simulink subsystem "Vehicle_Navigation"  (R2020b)
settings: Solver=VariableStepAuto  StartTime=0.0  StopTime=10.0  RelTol=1e-3
libraries: simulink_extras x1
settings Model: Creator=rthom  LastModifiedBy=david

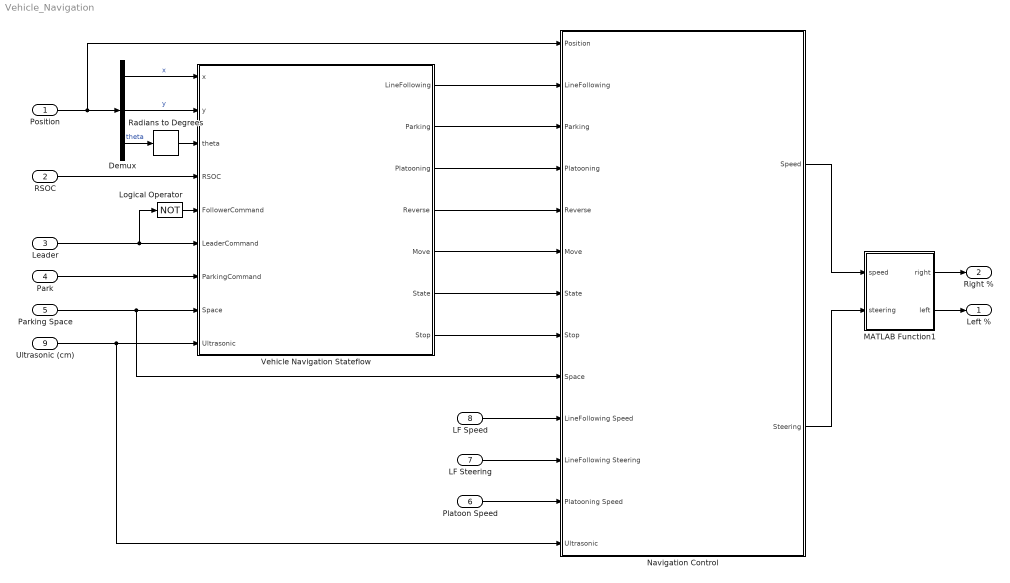
== system Vehicle_Navigation ==
  Position : Inport
  RSOC : Inport  Port=2
  Leader : Inport  Port=3
  Park : Inport  Port=4
  Parking Space : Inport  Port=5
  Platoon Speed : Inport  Port=6
  LF Steering : Inport  Port=7
  LF Speed : Inport  Port=8
  Ultrasonic (cm) : Inport  Port=9
  Demux : Demux  Outputs=3
  Logical Operator : Logic  Operator=NOT  AllPortsSameDT=off  OutDataTypeStr=boolean
  MATLAB Function1 : MATLAB Function  TreatAsAtomicUnit=on
  Navigation Control : Subsystem
  Radians to Degrees : simulink_extras/Transformations/Radians to Degrees
  Vehicle Navigation Stateflow : Stateflow chart  TreatAsAtomicUnit=on
  Left % : Outport
  Right % : Outport  Port=2
  wires:
  MATLAB Function1/1(right) -> Right %/1
  MATLAB Function1/2(left) -> Left %/1
  RSOC/1 -> Vehicle Navigation Stateflow/4(RSOC)
  Position/1 -> Demux/1, Navigation Control/1(Position)
  LF Speed/1 -> Navigation Control/10(LineFollowing Speed)
  Vehicle Navigation Stateflow/3(Platooning) -> Navigation Control/4(Platooning)
  Navigation Control/2(Steering) -> MATLAB Function1/2(steering)
  LF Steering/1 -> Navigation Control/11(LineFollowing Steering)
  Vehicle Navigation Stateflow/6(State) -> Navigation Control/7(State)
  Vehicle Navigation Stateflow/7(Stop) -> Navigation Control/8(Stop)
  Vehicle Navigation Stateflow/4(Reverse) -> Navigation Control/5(Reverse)
  Leader/1 -> Vehicle Navigation Stateflow/6(LeaderCommand), Logical Operator/1
  Vehicle Navigation Stateflow/1(LineFollowing) -> Navigation Control/2(LineFollowing)
  Vehicle Navigation Stateflow/2(Parking) -> Navigation Control/3(Parking)
  Demux/3 -> Radians to Degrees/1  "theta"
  Ultrasonic (cm)/1 -> Navigation Control/13(Ultrasonic), Vehicle Navigation Stateflow/9(Ultrasonic)
  Parking Space/1 -> Navigation Control/9(Space), Vehicle Navigation Stateflow/8(Space)
  Park/1 -> Vehicle Navigation Stateflow/7(ParkingCommand)
  Demux/2 -> Vehicle Navigation Stateflow/2(y)  "y"
  Platoon Speed/1 -> Navigation Control/12(Platooning Speed)
  Demux/1 -> Vehicle Navigation Stateflow/1(x)  "x"
  Vehicle Navigation Stateflow/5(Move) -> Navigation Control/6(Move)
  Navigation Control/1(Speed) -> MATLAB Function1/1(speed)
  Radians to Degrees/1 -> Vehicle Navigation Stateflow/3(theta)
  Logical Operator/1 -> Vehicle Navigation Stateflow/5(FollowerCommand)

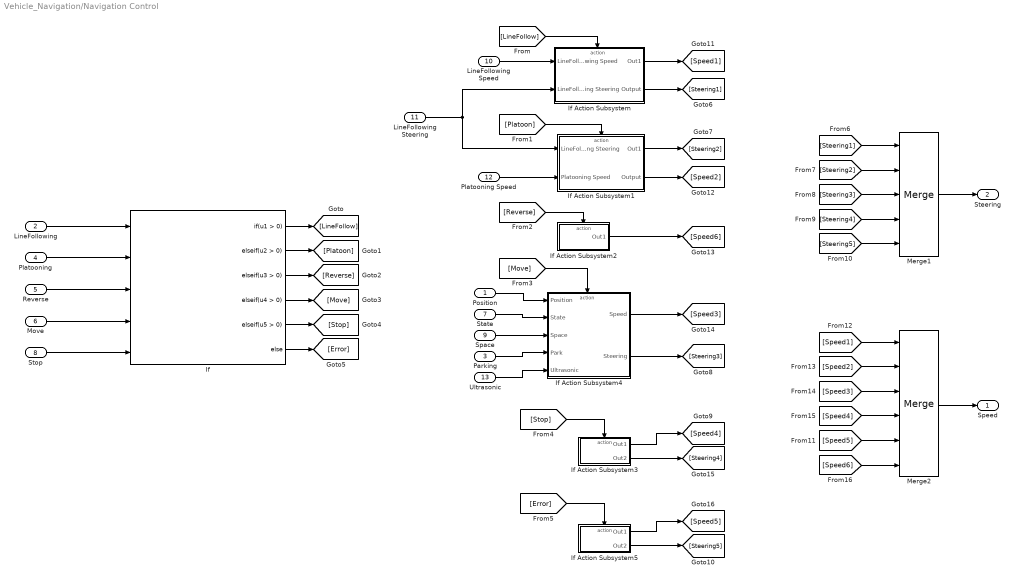
== system Vehicle_Navigation/Navigation Control ==
  Position : Inport
  LineFollowing : Inport  Port=2
  Parking : Inport  Port=3
  Platooning : Inport  Port=4
  Reverse : Inport  Port=5
  Move : Inport  Port=6
  State : Inport  Port=7
  Stop : Inport  Port=8
  Space : Inport  Port=9
  LineFollowing Speed : Inport  Port=10
  LineFollowing Steering : Inport  Port=11
  Platooning Speed : Inport  Port=12
  Ultrasonic : Inport  Port=13
  If : If  NumInputs=5  ElseIfExpressions=u2 > 0,u3 > 0,u4 > 0,u5 > 0
  If Action Subsystem : Subsystem  TreatAsAtomicUnit=on
  If Action Subsystem1 : Subsystem  TreatAsAtomicUnit=on
  If Action Subsystem2 : Subsystem  TreatAsAtomicUnit=on
  If Action Subsystem3 : Subsystem  TreatAsAtomicUnit=on
  If Action Subsystem4 : Subsystem  TreatAsAtomicUnit=on
  If Action Subsystem5 : Subsystem  TreatAsAtomicUnit=on
  Merge1 : Merge  Inputs=5
  Merge2 : Merge  Inputs=6
  Speed : Outport
  Steering : Outport  Port=2
  wires:
  Ultrasonic/1 -> If Action Subsystem4/5(Ultrasonic)
  Parking/1 -> If Action Subsystem4/4(Park)
  [Speed6] -> Merge2/6
  Merge2/1 -> Speed/1
  [Speed3] -> Merge2/3
  [Speed5] -> Merge2/5
  [Speed1] -> Merge2/1
  [Speed2] -> Merge2/2
  [Speed4] -> Merge2/4
  If Action Subsystem5/2(Out2) -> [Steering5]
  If Action Subsystem5/1(Out1) -> [Speed5]
  If Action Subsystem3/2(Out2) -> [Steering4]
  If Action Subsystem3/1(Out1) -> [Speed4]
  If Action Subsystem4/1(Speed) -> [Speed3]
  If Action Subsystem2/1(Out1) -> [Speed6]
  If Action Subsystem/1(Out1) -> [Speed1]
  [Steering5] -> Merge1/5
  [Steering4] -> Merge1/4
  [Steering3] -> Merge1/3
  If Action Subsystem4/2(Steering) -> [Steering3]
  Merge1/1 -> Steering/1
  [Steering2] -> Merge1/2
  [Steering1] -> Merge1/1
  If Action Subsystem/2(Output) -> [Steering1]
  LineFollowing Steering/1 -> If Action Subsystem1/1(LineFollowing Steering), If Action Subsystem/2(LineFollowing Steering)
  [Error] -> If Action Subsystem5/Action
  [Stop] -> If Action Subsystem3/Action
  [Move] -> If Action Subsystem4/Action
  [Reverse] -> If Action Subsystem2/Action
  [Platoon] -> If Action Subsystem1/Action
  Platooning Speed/1 -> If Action Subsystem1/2(Platooning Speed)
  [LineFollow] -> If Action Subsystem/Action
  If/6 -> [Error]
  If/5 -> [Stop]
  If/4 -> [Move]
  If/3 -> [Reverse]
  If/2 -> [Platoon]
  If/1 -> [LineFollow]
  LineFollowing Speed/1 -> If Action Subsystem/1(LineFollowing Speed)
  Space/1 -> If Action Subsystem4/3(Space)
  State/1 -> If Action Subsystem4/2(State)
  Position/1 -> If Action Subsystem4/1(Position)
  Stop/1 -> If/5
  Move/1 -> If/4
  Reverse/1 -> If/3
  Platooning/1 -> If/2
  LineFollowing/1 -> If/1
  If Action Subsystem1/2(Output) -> [Speed2]
  If Action Subsystem1/1(Out1) -> [Steering2]

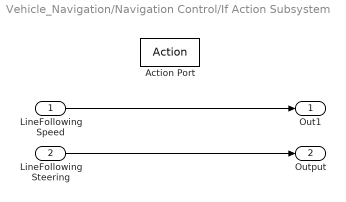
== system Vehicle_Navigation/Navigation Control/If Action Subsystem ==
  LineFollowing Speed : Inport
  LineFollowing Steering : Inport  Port=2
  Action Port : ActionPort
  Out1 : Outport
  Output : Outport  Port=2
  wires:
  LineFollowing Steering/1 -> Output/1
  LineFollowing Speed/1 -> Out1/1

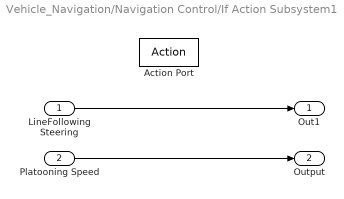
== system Vehicle_Navigation/Navigation Control/If Action Subsystem1 ==
  LineFollowing Steering : Inport
  Platooning Speed : Inport  Port=2
  Action Port : ActionPort
  Out1 : Outport
  Output : Outport  Port=2
  wires:
  Platooning Speed/1 -> Output/1
  LineFollowing Steering/1 -> Out1/1

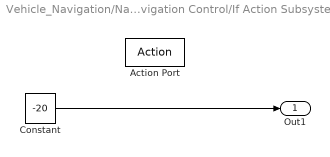
== system Vehicle_Navigation/Navigation Control/If Action Subsystem2 ==
  Action Port : ActionPort
  Constant : Constant  Value=-20
  Out1 : Outport
  wires:
  Constant/1 -> Out1/1

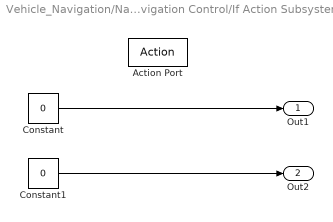
== system Vehicle_Navigation/Navigation Control/If Action Subsystem3 ==
  Action Port : ActionPort
  Constant : Constant  Value=0
  Constant1 : Constant  Value=0
  Out1 : Outport
  Out2 : Outport  Port=2
  wires:
  Constant1/1 -> Out2/1
  Constant/1 -> Out1/1

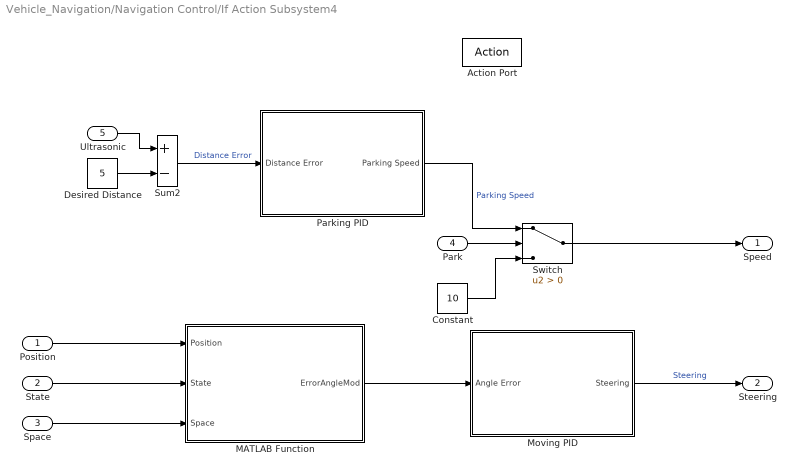
== system Vehicle_Navigation/Navigation Control/If Action Subsystem4 ==
  Position : Inport
  State : Inport  Port=2
  Space : Inport  Port=3
  Park : Inport  Port=4
  Ultrasonic : Inport  Port=5
  Action Port : ActionPort
  Constant : Constant  Value=10
  Desired Distance : Constant  Value=5
  MATLAB Function : MATLAB Function  TreatAsAtomicUnit=on
  Moving PID : Subsystem
  Parking PID : Subsystem
  Sum2 : Sum  Inputs=+-
  Switch : Switch  Criteria=u2 > Threshold
  Speed : Outport
  Steering : Outport  Port=2
  wires:
  Moving PID/1(Steering) -> Steering/1  "Steering"
  MATLAB Function/1(ErrorAngleMod) -> Moving PID/1(Angle Error)
  Parking PID/1(Parking Speed) -> Switch/1  "Parking Speed"
  Ultrasonic/1 -> Sum2/1
  Desired Distance/1 -> Sum2/2
  Sum2/1 -> Parking PID/1(Distance Error)  "Distance Error"
  Park/1 -> Switch/2
  Switch/1 -> Speed/1
  Constant/1 -> Switch/3
  Space/1 -> MATLAB Function/3(Space)
  State/1 -> MATLAB Function/2(State)
  Position/1 -> MATLAB Function/1(Position)

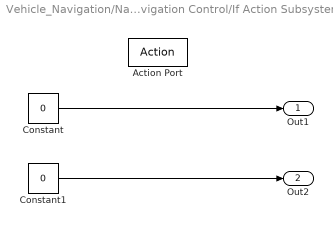
== system Vehicle_Navigation/Navigation Control/If Action Subsystem5 ==
  Action Port : ActionPort
  Constant : Constant  Value=0
  Constant1 : Constant  Value=0
  Out1 : Outport
  Out2 : Outport  Port=2
  wires:
  Constant1/1 -> Out2/1
  Constant/1 -> Out1/1

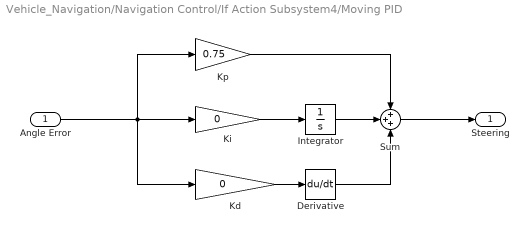
== system Vehicle_Navigation/Navigation Control/If Action Subsystem4/Moving PID ==
  Angle Error : Inport
  Derivative : Derivative
  Integrator : Integrator
  Kd : Gain  Gain=0
  Ki : Gain  Gain=0
  Kp : Gain  Gain=0.75
  Sum : Sum  Inputs=+++
  Steering : Outport
  wires:
  Derivative/1 -> Sum/3
  Angle Error/1 -> Kp/1, Ki/1, Kd/1
  Integrator/1 -> Sum/2
  Ki/1 -> Integrator/1
  Kp/1 -> Sum/1
  Kd/1 -> Derivative/1
  Sum/1 -> Steering/1

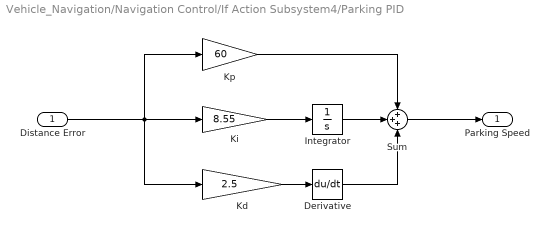
== system Vehicle_Navigation/Navigation Control/If Action Subsystem4/Parking PID ==
  Distance Error : Inport
  Derivative : Derivative
  Integrator : Integrator
  Kd : Gain  Gain=2.5
  Ki : Gain  Gain=8.55
  Kp : Gain  Gain=60
  Sum : Sum  Inputs=+++
  Parking Speed : Outport
  wires:
  Derivative/1 -> Sum/3
  Distance Error/1 -> Kp/1, Ki/1, Kd/1
  Integrator/1 -> Sum/2
  Ki/1 -> Integrator/1
  Kp/1 -> Sum/1
  Kd/1 -> Derivative/1
  Sum/1 -> Parking Speed/1

== matlab function Vehicle_Navigation/MATLAB Function1 ==
  data: right output; speed input; left output; steering input
function [right, left]= toMotorSpeeds(speed, steering)

left = speed - steering;
right = speed + steering;

m = max(left,right);
if m > 100
    left = left - m + 100;
    right = right - m + 100;
end

== matlab function Vehicle_Navigation/Navigation Control/If Action Subsystem4/MATLAB Function ==
  data: Position input; ErrorAngleMod output; State input; Space input
function ErrorAngleMod = NoLineFollowing(Position, State, Space)
%Define the desired angle depending on state and parking space requested
switch State
    case 3                              %State is exiting the track and moving towards the staging area.
        if Space == 3                       %Staging area set for parking space 1
            Dist_Z = 1.8 - Position(2);         %Z distance between vehicle and staging area
            Dist_X = 0 - Position(1);           %X distance betweeen vehicle and staging area
        elseif Space == 2                   %Staging area set for parking space 2
            Dist_Z = 1.5 - Position(2);       %Z distance between vehicle and staging area
            Dist_X = 0 - Position(1);           %X distance between vehicle and staging area
        else                                %Staging area set for parking space 3
            Dist_Z = 1.1 - Position(2);         %Z distance between vehicle and staging area
            Dist_X = 0 - Position(1);           %X distance between vehicle and staging area
        end
        DesiredAngle = atan2(Dist_Z,Dist_X); %Calculate the desired trajectory angle
        
    case 4                              %State is moving to the parking space
        if Space == 3                       %Set for parking space 1
            Dist_Z = 1.6 - Position(2);         %Z distance between vehicle and parking spot
            Dist_X = -0.45 - Position(1);       %X distance betweeen vehicle and parking spot
        elseif Space == 2                   %Set for parking space 2
            Dist_Z = 1.2 - Position(2);         %Z distance between vehicle and parking spot
            Dist_X = -0.75 - Position(1);       %X distance between vehicle and parking spot
        else                                %Set for parking space 3
            Dist_Z = 0.8 - Position(2);         %Z distance between vehicle and parking spot
            Dist_X = -0.85 - Position(1);       %X distance between vehicle and parking spot
        end
        DesiredAngle = atan2(Dist_Z,Dist_X); %Calculate the desired trajectory angle
        
    case 5                              %State is moving into the parking space
        DesiredAngle = pi;                  %Angle set to 180 degrees
        
    case 9                              %State is moving to the stop sign
        Dist_Z = 0.525 - Position(2);       %Z distance between vehicle and parking spot
        Dist_X = 0.0935 - Position(1);      %X distance between vehicle and parking spot
        DesiredAngle = atan2(Dist_Z,Dist_X); %Calculate the desired trajectory angle

    case 10                              %State is moving to the stop sign
        if Space == 3                       %Staging area set for parking space 1
            Dist_Z = 0.26 - Position(2);         %Z distance between vehicle and staging area
            Dist_X = -0.27 - Position(1);           %X distance betweeen vehicle and staging area
        elseif Space == 2                   %Staging area set for parking space 2
            Dist_Z = 0.26 - Position(2);       %Z distance between vehicle and staging area
            Dist_X = -0.63 - Position(1);           %X distance between vehicle and staging area
        else                                %Staging area set for parking space 3
            Dist_Z = 0.26 - Position(2);         %Z distance between vehicle and staging area
            Dist_X = -1.0 - Position(1);           %X distance between vehicle and staging area
        end
        DesiredAngle = atan2(Dist_Z,Dist_X); %Calculate the desired trajectory angle
%         Dist_Z = 0.33 - Position(2);        %Z distance between vehicle and parking spot
%         Dist_X = -0.3 - Position(1);        %X distance between vehicle and parking spot
%         DesiredAngle = atan2(Dist_Z,Dist_X); %Calculate the desired trajectory angle
    
    case 11                              %State is moving into the parking space
        DesiredAngle = pi;                  %Angle set to 180 degrees
        
    otherwise
        DesiredAngle = 0;
end

%Calculate Error for PID controller
DesiredAngle = rad2deg(DesiredAngle);
ActualAngle = rad2deg(Position(3));

ErrorAngle = DesiredAngle - ActualAngle;

ErrorAngleMod = mod(ErrorAngle + 180, 360) - 180;
end

== stateflow chart Vehicle_Navigation/Vehicle Navigation Stateflow ==
  state IsLeader
    %EV is set as the leader
    entry:
    LineFollowing = 1;%Line Following enabled
    Platooning = 0;%Platooning disabled
    Stop = 0;%Stopping disabled
    Reverse = 0;%Reversing disabled
    Move = 0;%Non-line following movement disabled
    Parking = 0;%Parking using ultrasonic sensor disabled
    State = 0;
  state IsFindingParking
    %EV rotates and moves toward parking position.
    entry:
    LineFollowing = 0;%Line Following disabled
    Platooning = 0;%Platooning disabled
    Stop = 0;%Stopping disabled
    Reverse = 0;%Reversing disabled
    Move = 1;%Movement towards parking.
    Parking = 0;%Parking using ultrasonic sensor disabled
    State = 4;
  state IsParkingIntoSpace
    %EV rotates and moves toward parking position
    %using the ultrasonic sensor in parking mode.
    entry:
    LineFollowing = 0;%Line Following disabled
    Platooning = 0;%Platooning disabled
    Stop = 0;%Stopping disabled
    Reverse = 0;%Reversing disabled
    Move = 1;%Move perpendicular to the spot
    Parking = 1;%Parking using ultrasonic sensor enabled
    State = 5;
  state IsStopped
    %EV moves to the desired distance away from the
    %front of the parking space
    entry:
    LineFollowing = 0;%Line Following disabled
    Platooning = 0;%Platooning disabled
    Stop = 1;%Stopping enabled
    Reverse = 0;%Reversing disabled
    Move = 0;%Movement disabled
    Parking = 0;%Parking using ultrasonic sensor disabled
    State = 6;
  state IsReversing
    %EV reverses out of parking spot and stages.
    entry:
    LineFollowing = 0;%Line Following disabled
    Platooning = 0;%Platooning disabled
    Stop = 0;%Stopping disabled
    Reverse = 1;%Reversing enabled
    Move = 0;%Movement disabled
    Parking = 0;%Parking using ultrasonic sensor disabled
    State = 7;
  state IsGoToStopSign
    %EV moves to the stop sign
    entry:
    LineFollowing = 0;%Line Following disabled
    Platooning = 0;%Platooning disabled
    Stop = 0;%Stopping disabled
    Reverse = 0;%Reversing disabled
    Move = 1;%Move towards the stop sign
    Parking = 0;%Parking using ultrasonic sensor disabled
    State = 9;
  state IsEnteringTrack
    %EV moves to the track entrance, enters track, and
    %rotates in the correct orientation.
    entry:
    LineFollowing = 0;%Line Following disabled
    Platooning = 0;%Platooning disabled
    Stop = 0;%Stopping disabled
    Reverse = 0;%Reversing disabled
    Move = 1;%Move onto the track
    Parking = 0;%Parking using ultrasonic sensor disabled
    State = 10;
  state IsRotate
    %EV moves to the track entrance, enters track, and
    %rotates in the correct orientation.
    entry:
    LineFollowing = 0;%Line Following disabled
    Platooning = 0;%Platooning disabled
    Stop = 0;%Stopping disabled
    Reverse = 0;%Reversing disabled
    Move = 1;%Move onto the track
    Parking = 0;%Parking using ultrasonic sensor disabled
    State = 11;
  state IsExitingTrack
    %EV reaches exit ramp and stops
    %using the line following and
    %platooning controllers, rotates
    %towards the parking area, then moves to staging .
    entry:
    LineFollowing = 0;%Line Following disabled
    Platooning = 0;%Platooning disabled
    Stop = 0;%Stopping disabled
    Reverse = 0;%Reverse disabled
    Move = 1;%Movement enabled, Towards staging area
    State = 3;
  state IsParking
    %EV is told to park and initializes
    %assocaited values. If the EV
    %reaches the ramp it moves to next
    %state. If parking button pressed
    %again, it will return to either leader
    %or follower state.
    entry:
    Stop = 0;%Stoping disabled
    Reverse = 0;%Reverse disabled
    Move = 0;%Non-line following movement disabled
    State = 2;
  state IsFollower
    %EV is set as the follower
    entry:
    LineFollowing = 0;%Line Following disabled
    Platooning = 1;%Platooning enabled (includes line following)
    Stop = 0;%Stopping disabled
    Reverse = 0;%Reversing disabled
    Move = 0;%Non-line following movement disabled
    Parking = 0;%Parking using ultrasonic sensor disabled
    State = 1;
  IsRotate -> IsLeader [order 1] : [LeaderCommand == 1 &&...
      | (mod(theta,180) >= -1 && mod(theta,180) <= 1)]
  (default) -> IsLeader
  IsParking -> IsLeader [order 2] : [ParkingCommand == 0 && ...
      | LeaderCommand ==1]
  IsLeader -> IsParking [order 2] : [ParkingCommand == 1]
  IsFollower -> IsLeader [order 1] : [LeaderCommand == 1]
  IsLeader -> IsFollower [order 1] : [FollowerCommand == 1]
  IsParking -> IsExitingTrack [order 1] : [(x <= 0.2 && x >= -0.2)...
      | && (y <= 3 && y >= 2)]
  IsStopped -> IsReversing : [RSOC == 100 ||...
      | ParkingCommand == 0]
  IsExitingTrack -> IsFindingParking : [((Space == 3 && (x >= -0.3 && x <= 0.3) && (y >= 1.7 && y <= 1.9)) ||...
      | (Space == 2 &&  (x >= -0.3 && x <= 0.3) && (y >= 1.4 && y <= 1.6)) ||...
      | (Space == 1 &&  (x >= -0.3 && x <= 0.3) && (y >= 1.0 && y <= 1.2)))]
  IsGoToStopSign -> IsEnteringTrack : [(x >= 0.017 & x <= 0.17) &&...
      | (y >= 0.45 && y <= 0.6)]
  IsReversing -> IsGoToStopSign : [((Space == 3 && (x >= -0.3 && x <= 0.3) && (y >= 1.4 && y <= 1.9)) ||...
      | (Space == 2 &&  (x >= -0.3 && x <= 0.3) && (y >= 1.0 && y <= 1.5)) ||...
      | (Space == 1 &&  (x >= -0.3 && x <= 0.3) && (y >= 0.6 && y <= 1.3)))]
  IsFindingParking -> IsParkingIntoSpace : [((Space == 3 && (x >= -0.5 && x <= -0.4) && (y >= 1.5 && y <= 1.7)) ||...
      | (Space == 2 &&  (x >= -0.8 && x <= -0.7) && (y >= 1.1 && y <= 1.3)) ||...
      | (Space == 1 &&  (x >= -0.9 && x <= -0.8) && (y >= 0.7 && y <= 0.9)))]
  IsParkingIntoSpace -> IsStopped : [((Space == 3 && (x >= -0.6 && x <= -0.5) && (y >= 1.5 && y <= 1.7)) ||...
      | (Space == 2 &&  (x >= -0.9 && x <= -0.8) && (y >= 1.1 && y <= 1.3)) ||...
      | (Space == 1 &&  (x >= -1.0 && x <= -0.9) && (y >= 0.7 && y <= 0.9)))]
  IsEnteringTrack -> IsRotate : [((Space == 3 && (x >= -0.28 && x <= -0.26) && (y >= 0.25 && y <= 0.27)) ||...
      | (Space == 2 &&  (x >= -0.64 && x <= -0.62) && (y >= 0.25 && y <= 0.27)) ||...
      | (Space == 1 &&  (x >= -1.1 && x <= -0.9) && (y >= 0.25 && y <= 0.27)))]
  IsFollower -> IsParking [order 2] : [ParkingCommand == 1]
  IsParking -> IsFollower [order 3] : [ParkingCommand == 0 && ...
      | FollowerCommand == 1]
  IsRotate -> IsFollower [order 2] : [FollowerCommand == 1 &&...
      | mod(theta,180) == 0]
  data: x input; y input; theta input; RSOC input; FollowerCommand input; LeaderCommand input; ParkingCommand input; Space input; Ultrasonic input; LineFollowing output; Parking output; Platooning output; Reverse output; Move output; State output; Stop output
